simulink model "Assignment2"  (R2021a)
settings: Solver=FixedStepAuto  StartTime=0.0  StopTime=2  FixedStep=1e-3  RelTol=1e-3  EnableMultiTasking=on
undefined symbols (not defined in the file): D0, D1, D10, D11, D12, D13, D2, D3, D4, D5, D6, D7, D8, D9, magnitude, PTA0, PTA1, PTA2, PTB23, PTB9, PTC16, PTC17, PTC2, PTC3, PTC4, PTD0, PTD1, PTD2, PTD3
libraries: frdmk64flib x19, dspstat3 x1
settings Model: EnablePacing=on  PacingRate=0.250000  ExtModeTrigDuration=5  Creator=Arun Mistry  LastModifiedBy=majet
settings OptimizationCC: EnhancedBackFolding=on  PassReuseOutputArgsAs=Individual arguments  ZeroExternalMemoryAtStartup=off  ZeroInternalMemoryAtStartup=off  MaxStackSize=64  OptimizeBlockOrder=speed  DifferentSizesBufferReuse=on  OptimizationCustomize=off  EfficientTunableParamExpr=on
settings DebuggingCC: ParameterTunabilityLossMsg=error
settings HardwareCC: ProdBitPerPointer=32  ProdBitPerSizeT=32  ProdBitPerPtrDiffT=32  ProdLargestAtomicInteger=Long  ProdLargestAtomicFloat=Double  ProdWordSize=32  ProdHWDeviceType=ARM Compatible->ARM Cortex
settings SFSimCC: MATLABDynamicMemAlloc=off
settings RTWCC: SystemTargetFile=ert.tlc  HardwareBoard=NXP FRDM-K64F  TLCOptions="-aInlineSetEventsForThisBaseRateFcn=TLC_FALSE -aSuppressMultiTaskScheduler=TLC_FALSE  -aRateBasedStepFcn=0"  TemplateMakefile=ert_default_tmf  Toolchain=GNU Tools for ARM Embedded Processors
settings CodeAppCC: ForceParamTrailComments=on  IgnoreCustomStorageClasses=off  OperatorAnnotations=on  SimulinkDataObjDesc=on  SFDataObjDesc=on  InsertBlockDesc=on
settings ERTTargetCC: ExtModeTransport=4  ExtModeMexFile=sendToCommService

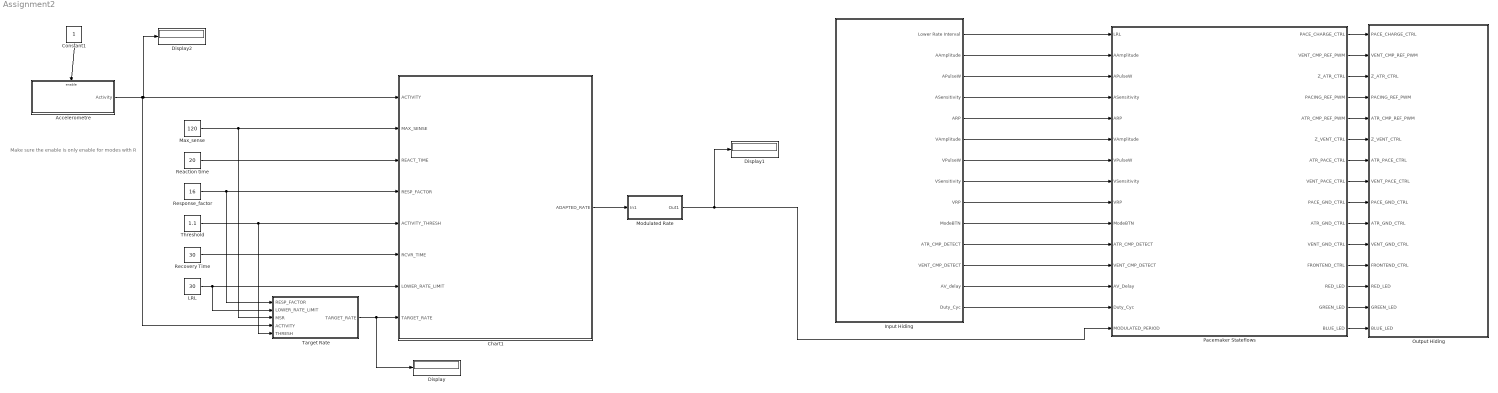
== system Assignment2 ==
  note: Make sure the enable is only enable for modes with R
  Accelerometre : Subsystem
  Chart1 : Stateflow chart  TreatAsAtomicUnit=on
  Constant1 : Constant  OutDataTypeStr=uint16
  Display : Display
  Display1 : Display
  Display2 : Display
  Input Hiding : Subsystem
  LRL : Constant  Value=30  OutDataTypeStr=uint16
  Max_sense : Constant  Value=120  OutDataTypeStr=uint16
  Modulated Rate : Subsystem
  Output Hiding : Subsystem
  Pacemaker Stateflows : Stateflow chart  TreatAsAtomicUnit=on
      settings: PortSchema="{\"entries\":[{\"content\":{\"sides\":[{\"content\":{\"connectorIds\":[\"In1\",\"In2\",\"In3\",\"In4\",\"In5\",\"In6\",\"In7\",\"In8\",\"In9\",\"In10\",\"In11\",\"In12\",\"In13\",\"In15\",\"In14\"]},\"type\":\"ConnectorPlacement.EquallySpacedRectSide\",\"uuid\":\"73ec282f-bdc5-469f-8e6f-a94c3bdc9020\"},{\"content\":{\"connectorIds\":[\"Out1\",\"Out2\",\"Out3\",\"Out4\",\"Out5\",\"Out6\",\"Out7\",\"Out8\",\"Out9\",\"Out10\",\"Out11\",\"Out12\",\"Out13\",\"Out14\",\"Out15\"],\"side\":\"RIGHT\"},\"type\":\"ConnectorPlacement.EquallySpacedRectSide\",\"uuid\":\"8dd20006-a4c5-4baa-83a8-987332cd4bb4\"},{\"content\":{\"connectorIds\":[],\"side\":\"TOP\"},\"type\":\"ConnectorPlacement.EquallySpacedRectSide\",\"uuid\":\"22935e9b-efaa-43e1-8cc8-2e08fa14d9a6\"},{\"content\":{\"connectorIds\":[],\"side\":\"BOTTOM\"},\"type\":\"ConnectorPlacement.EquallySpacedRectSide\",\"uuid\":\"9851d334-d076-4ac0-89c9-77644970121a\"}]},\"type\":\"ConnectorPlacement.EquallySpacedConnector\",\"uuid\":\"2847227f-03fa-454f-95d6-41e472bd469d\"}],\"packageUris\":[\"http://schema.mathworks.com/mf0/Connector/R2020b\"],\"version\":\"1.0\"}"
  Reaction time : Constant  Value=20  OutDataTypeStr=uint16
  Recovery Time : Constant  Value=30  OutDataTypeStr=uint16
  Response_factor : Constant  Value=16  OutDataTypeStr=uint16
  Target Rate : Subsystem
  Threshold : Constant  Value=1.1  OutDataTypeStr=double
  wires:
  Pacemaker Stateflows/1(PACE_CHARGE_CTRL) -> Output Hiding/1(PACE_CHARGE_CTRL)
  Input Hiding/11(ATR_CMP_DETECT) -> Pacemaker Stateflows/11(ATR_CMP_DETECT)
  Input Hiding/7(VPulseW) -> Pacemaker Stateflows/7(VPulseW)
  Input Hiding/12(VENT_CMP_DETECT) -> Pacemaker Stateflows/12(VENT_CMP_DETECT)
  Pacemaker Stateflows/3(Z_ATR_CTRL) -> Output Hiding/3(Z_ATR_CTRL)
  Input Hiding/3(APulseW) -> Pacemaker Stateflows/3(APulseW)
  Pacemaker Stateflows/7(ATR_PACE_CTRL) -> Output Hiding/7(ATR_PACE_CTRL)
  Pacemaker Stateflows/10(ATR_GND_CTRL) -> Output Hiding/10(ATR_GND_CTRL)
  Input Hiding/10(ModeBTN) -> Pacemaker Stateflows/10(ModeBTN)
  Input Hiding/2(AAmplitude) -> Pacemaker Stateflows/2(AAmplitude)
  Input Hiding/6(VAmplitude) -> Pacemaker Stateflows/6(VAmplitude)
  Pacemaker Stateflows/6(Z_VENT_CTRL) -> Output Hiding/6(Z_VENT_CTRL)
  Pacemaker Stateflows/4(PACING_REF_PWM) -> Output Hiding/4(PACING_REF_PWM)
  Pacemaker Stateflows/11(VENT_GND_CTRL) -> Output Hiding/11(VENT_GND_CTRL)
  Pacemaker Stateflows/9(PACE_GND_CTRL) -> Output Hiding/9(PACE_GND_CTRL)
  Pacemaker Stateflows/8(VENT_PACE_CTRL) -> Output Hiding/8(VENT_PACE_CTRL)
  Input Hiding/1(Lower Rate Interval) -> Pacemaker Stateflows/1(LRL)
  Pacemaker Stateflows/15(BLUE_LED) -> Output Hiding/15(BLUE_LED)
  Input Hiding/4(ASensitivity) -> Pacemaker Stateflows/4(ASensitivity)
  Pacemaker Stateflows/12(FRONTEND_CTRL) -> Output Hiding/12(FRONTEND_CTRL)
  Input Hiding/9(VRP) -> Pacemaker Stateflows/9(VRP)
  Input Hiding/8(VSensitivity) -> Pacemaker Stateflows/8(VSensitivity)
  Input Hiding/5(ARP) -> Pacemaker Stateflows/5(ARP)
  Pacemaker Stateflows/14(GREEN_LED) -> Output Hiding/14(GREEN_LED)
  Pacemaker Stateflows/13(RED_LED) -> Output Hiding/13(RED_LED)
  Pacemaker Stateflows/5(ATR_CMP_REF_PWM) -> Output Hiding/5(ATR_CMP_REF_PWM)
  Pacemaker Stateflows/2(VENT_CMP_REF_PWM) -> Output Hiding/2(VENT_CMP_REF_PWM)
  Input Hiding/14(Duty_Cyc) -> Pacemaker Stateflows/15(Duty_Cyc)
  LRL/1 -> Target Rate/2(LOWER_RATE_LIMIT), Chart1/7(LOWER_RATE_LIMIT)
  Chart1/1(ADAPTED_RATE) -> Modulated Rate/1(In1)
  Recovery Time/1 -> Chart1/6(RCVR_TIME)
  Max_sense/1 -> Target Rate/3(MSR), Chart1/2(MAX_SENSE)
  Reaction time/1 -> Chart1/3(REACT_TIME)
  Response_factor/1 -> Target Rate/1(RESP_FACTOR), Chart1/4(RESP_FACTOR)
  Threshold/1 -> Target Rate/5(THRESH), Chart1/5(ACTIVITY_THRESH)
  Modulated Rate/1(Out1) -> Display1/1, Pacemaker Stateflows/14(MODULATED_PERIOD)
  Constant1/1 -> Accelerometre/Enable
  Input Hiding/13(AV_delay) -> Pacemaker Stateflows/13(AV_Delay)
  Target Rate/1(TARGET_RATE) -> Display/1, Chart1/8(TARGET_RATE)
  Accelerometre/1(Activity) -> Target Rate/4(ACTIVITY), Chart1/1(ACTIVITY), Display2/1

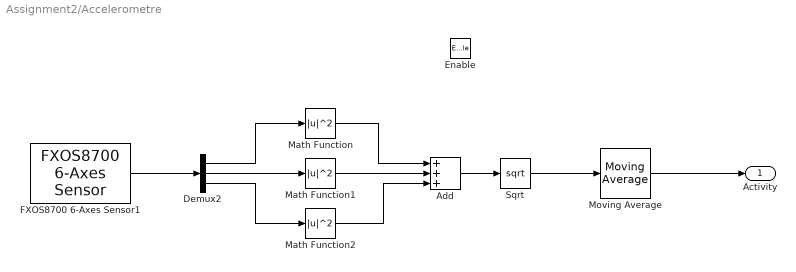
== system Assignment2/Accelerometre ==
  Enable : EnablePort
  Add : Sum  Inputs=+++
  Demux2 : Demux  Outputs=3
  FXOS8700 6-Axes Sensor1 : frdmk64flib/FXOS8700 6-Axes Sensor  Activesensor=Accelerometer only  ODR=100Hz  HybridODR=400Hz  Accelfullrange=-4g to +4g  SampleTime=1/100
  Math Function : Math  Operator=magnitude^2  SignedPower=on  OutDataTypeStr=double  SaturateOnIntegerOverflow=on
  Math Function1 : Math  Operator=magnitude^2  SignedPower=on  OutDataTypeStr=double  SaturateOnIntegerOverflow=on
  Math Function2 : Math  Operator=magnitude^2  SignedPower=on  OutDataTypeStr=double  SaturateOnIntegerOverflow=on
  Moving Average : dspstat3/Moving Average  Method=Sliding window  ForgettingFactorPort=off  SpecifyWindowLength=on  WindowLength=4  ForgettingFactor=0.9  SimulateUsing=Code generation
  Sqrt : Sqrt  SaturateOnIntegerOverflow=on
  Activity : Outport  OutDataTypeStr=double  SourceOfInitialOutputValue=Input signal
  wires:
  Sqrt/1 -> Moving Average/1
  FXOS8700 6-Axes Sensor1/1 -> Demux2/1
  Math Function/1 -> Add/1
  Add/1 -> Sqrt/1
  Math Function2/1 -> Add/3
  Demux2/2 -> Math Function1/1
  Math Function1/1 -> Add/2
  Demux2/1 -> Math Function/1
  Demux2/3 -> Math Function2/1
  Moving Average/1 -> Activity/1

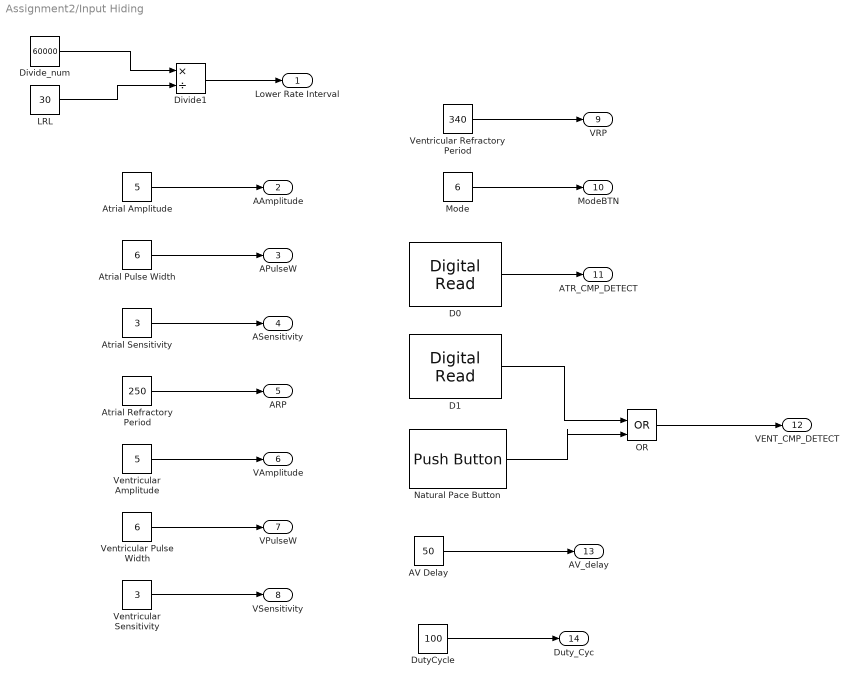
== system Assignment2/Input Hiding ==
  AV Delay : Constant  Value=50  OutDataTypeStr=uint16
  Atrial Amplitude : Constant  Value=5  OutDataTypeStr=uint16
  Atrial Pulse Width : Constant  Value=6  OutDataTypeStr=uint16
  Atrial Refractory Period : Constant  Value=250  OutDataTypeStr=uint16
  Atrial Sensitivity : Constant  Value=3  OutDataTypeStr=uint16
  D0 : frdmk64flib/Digital Read  Whichpin=PTC16 (D0)  SampleTime=-1
  D1 : frdmk64flib/Digital Read  Whichpin=PTC17 (D1)  SampleTime=-1
  Divide1 : Product  Inputs=*/  OutDataTypeStr=uint16  RndMeth=Round
  Divide_num : Constant  Value=60000  OutDataTypeStr=uint16
  DutyCycle : Constant  Value=100  OutDataTypeStr=uint16
  LRL : Constant  Value=30  OutDataTypeStr=uint16
  Mode : Constant  Value=6  OutDataTypeStr=uint16
  Natural Pace Button : frdmk64flib/Push Button  Whichswitch=SW3  SampleTime1=-1
  OR : Logic  Operator=OR  IconShape=distinctive  AllPortsSameDT=off  OutDataTypeStr=boolean
  Ventricular Amplitude : Constant  Value=5  OutDataTypeStr=uint16
  Ventricular Pulse Width : Constant  Value=6  OutDataTypeStr=uint16
  Ventricular Refractory Period : Constant  Value=340  OutDataTypeStr=uint16
  Ventricular Sensitivity : Constant  Value=3  OutDataTypeStr=uint16
  Lower Rate Interval : Outport  OutDataTypeStr=uint16
  AAmplitude : Outport  Port=2  OutDataTypeStr=uint16
  APulseW : Outport  Port=3  OutDataTypeStr=uint16
  ASensitivity : Outport  Port=4  OutDataTypeStr=uint16
  ARP : Outport  Port=5  OutDataTypeStr=uint16
  VAmplitude : Outport  Port=6  OutDataTypeStr=uint16
  VPulseW : Outport  Port=7  OutDataTypeStr=uint16
  VSensitivity : Outport  Port=8  OutDataTypeStr=uint16
  VRP : Outport  Port=9  OutDataTypeStr=uint16
  ModeBTN : Outport  Port=10  OutDataTypeStr=uint16
  ATR_CMP_DETECT : Outport  Port=11  OutDataTypeStr=boolean
  VENT_CMP_DETECT : Outport  Port=12  OutDataTypeStr=boolean
  AV_delay : Outport  Port=13  OutDataTypeStr=uint16
  Duty_Cyc : Outport  Port=14  OutDataTypeStr=uint16
  wires:
  Atrial Amplitude/1 -> AAmplitude/1
  Ventricular Amplitude/1 -> VAmplitude/1
  Atrial Pulse Width/1 -> APulseW/1
  Ventricular Pulse Width/1 -> VPulseW/1
  Atrial Sensitivity/1 -> ASensitivity/1
  Ventricular Sensitivity/1 -> VSensitivity/1
  Ventricular Refractory Period/1 -> VRP/1
  Atrial Refractory Period/1 -> ARP/1
  D0/1 -> ATR_CMP_DETECT/1
  Natural Pace Button/1 -> OR/2
  Mode/1 -> ModeBTN/1
  DutyCycle/1 -> Duty_Cyc/1
  Divide_num/1 -> Divide1/1
  Divide1/1 -> Lower Rate Interval/1
  D1/1 -> OR/1
  OR/1 -> VENT_CMP_DETECT/1
  AV Delay/1 -> AV_delay/1
  LRL/1 -> Divide1/2

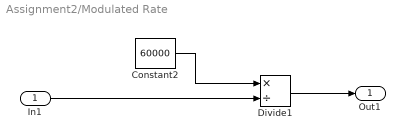
== system Assignment2/Modulated Rate ==
  In1 : Inport  OutDataTypeStr=uint16
  Constant2 : Constant  Value=60000  OutDataTypeStr=uint16
  Divide1 : Product  Inputs=*/  OutDataTypeStr=uint16
  Out1 : Outport  OutDataTypeStr=uint16
  wires:
  In1/1 -> Divide1/2
  Constant2/1 -> Divide1/1
  Divide1/1 -> Out1/1

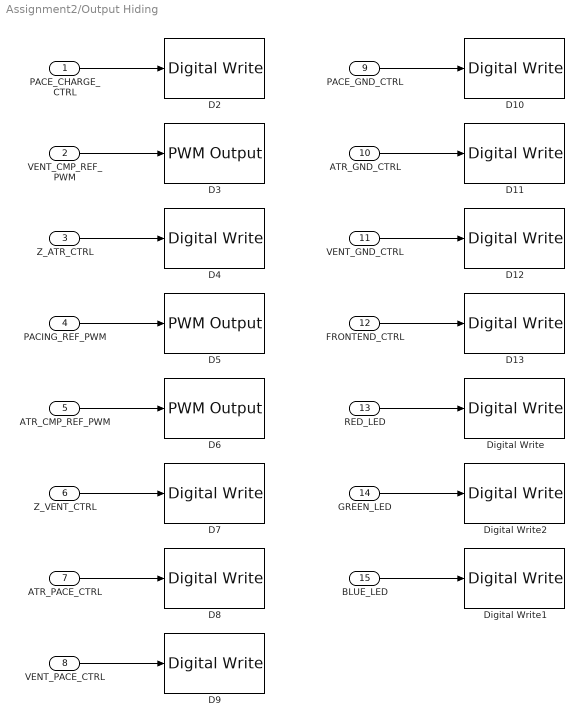
== system Assignment2/Output Hiding ==
  PACE_CHARGE_CTRL : Inport  OutDataTypeStr=uint16
  VENT_CMP_REF_PWM : Inport  Port=2  OutDataTypeStr=uint16
  Z_ATR_CTRL : Inport  Port=3  OutDataTypeStr=uint16
  PACING_REF_PWM : Inport  Port=4  OutDataTypeStr=uint16
  ATR_CMP_REF_PWM : Inport  Port=5  OutDataTypeStr=uint16
  Z_VENT_CTRL : Inport  Port=6  OutDataTypeStr=uint16
  ATR_PACE_CTRL : Inport  Port=7  OutDataTypeStr=uint16
  VENT_PACE_CTRL : Inport  Port=8  OutDataTypeStr=uint16
  PACE_GND_CTRL : Inport  Port=9  OutDataTypeStr=uint16
  ATR_GND_CTRL : Inport  Port=10  OutDataTypeStr=uint16
  VENT_GND_CTRL : Inport  Port=11  OutDataTypeStr=uint16
  FRONTEND_CTRL : Inport  Port=12  OutDataTypeStr=uint16
  RED_LED : Inport  Port=13  OutDataTypeStr=uint16
  GREEN_LED : Inport  Port=14  OutDataTypeStr=uint16
  BLUE_LED : Inport  Port=15  OutDataTypeStr=uint16
  D10 : frdmk64flib/Digital Write  Whichpin=PTD0 (D10)
  D11 : frdmk64flib/Digital Write  Whichpin=PTD2 (D11)
  D12 : frdmk64flib/Digital Write  Whichpin=PTD3 (D12)
  D13 : frdmk64flib/Digital Write  Whichpin=PTD1 (D13)
  D2 : frdmk64flib/Digital Write  Whichpin=PTB9 (D2)
  D3 : frdmk64flib/PWM Output  Whichpin=PTA1 (D3)  InitialFrequency=2000  InitialDutyCycle=100
  D4 : frdmk64flib/Digital Write  Whichpin=PTB23 (D4)
  D5 : frdmk64flib/PWM Output  Whichpin=PTA2 (D5)  InitialFrequency=2000  InitialDutyCycle=100
  D6 : frdmk64flib/PWM Output  Whichpin=PTC2 (D6)  InitialFrequency=2000  InitialDutyCycle=100
  D7 : frdmk64flib/Digital Write  Whichpin=PTC3 (D7)
  "D8 " : frdmk64flib/Digital Write  Whichpin=PTA0 (D8)
  D9 : frdmk64flib/Digital Write  Whichpin=PTC4 (D9)
  Digital Write : frdmk64flib/Digital Write  Whichpin=RED_LED
  Digital Write1 : frdmk64flib/Digital Write  Whichpin=BLUE_LED
  Digital Write2 : frdmk64flib/Digital Write  Whichpin=GREEN_LED
  wires:
  VENT_PACE_CTRL/1 -> D9/1
  ATR_CMP_REF_PWM/1 -> D6/1
  PACE_GND_CTRL/1 -> D10/1
  VENT_CMP_REF_PWM/1 -> D3/1
  PACING_REF_PWM/1 -> D5/1
  ATR_GND_CTRL/1 -> D11/1
  ATR_PACE_CTRL/1 -> "D8 "/1
  PACE_CHARGE_CTRL/1 -> D2/1
  FRONTEND_CTRL/1 -> D13/1
  VENT_GND_CTRL/1 -> D12/1
  Z_ATR_CTRL/1 -> D4/1
  Z_VENT_CTRL/1 -> D7/1
  RED_LED/1 -> Digital Write/1
  BLUE_LED/1 -> Digital Write1/1
  GREEN_LED/1 -> Digital Write2/1

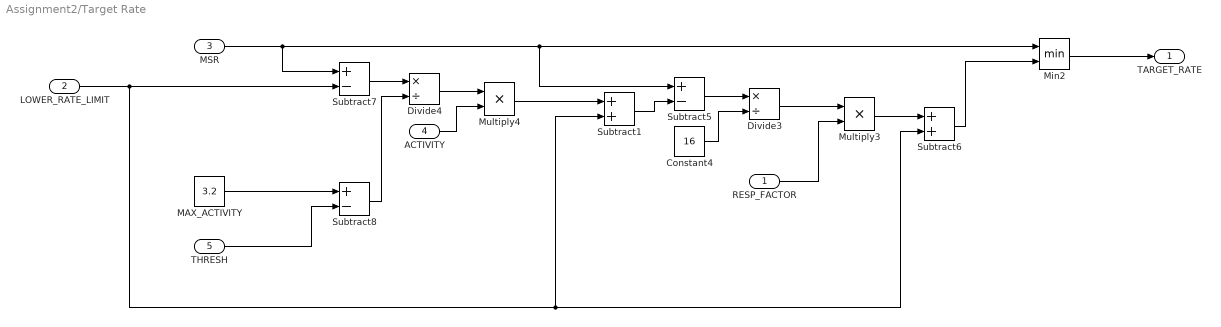
== system Assignment2/Target Rate ==
  RESP_FACTOR : Inport  OutDataTypeStr=uint16
  LOWER_RATE_LIMIT : Inport  Port=2  OutDataTypeStr=uint16
  MSR : Inport  Port=3  OutDataTypeStr=uint16
  ACTIVITY : Inport  Port=4  OutDataTypeStr=double
  THRESH : Inport  Port=5  OutDataTypeStr=double
  Constant4 : Constant  Value=16  OutDataTypeStr=double
  Divide3 : Product  Inputs=*/  OutDataTypeStr=uint16
  Divide4 : Product  Inputs=*/  OutDataTypeStr=uint16
  MAX_ACTIVITY : Constant  Value=3.2  OutDataTypeStr=double
  Min2 : MinMax  Inputs=2
  Multiply3 : Product  Inputs=**  OutDataTypeStr=uint16  RndMeth=Ceiling
  Multiply4 : Product  Inputs=**  OutDataTypeStr=uint16  RndMeth=Ceiling
  Subtract1 : Sum  AccumDataTypeStr=uint16
  Subtract5 : Sum  Inputs=+-  AccumDataTypeStr=uint16
  Subtract6 : Sum  AccumDataTypeStr=uint16
  Subtract7 : Sum  Inputs=+-  AccumDataTypeStr=uint16
  Subtract8 : Sum  Inputs=+-  AccumDataTypeStr=double
  TARGET_RATE : Outport  OutDataTypeStr=uint16  SourceOfInitialOutputValue=Input signal
  wires:
  MSR/1 -> Subtract5/1, Min2/1, Subtract7/1
  ACTIVITY/1 -> Multiply4/2
  Constant4/1 -> Divide3/2
  Divide4/1 -> Multiply4/1
  Divide3/1 -> Multiply3/1
  Subtract5/1 -> Divide3/1
  MAX_ACTIVITY/1 -> Subtract8/1
  Subtract6/1 -> Min2/2
  Subtract8/1 -> Divide4/2
  LOWER_RATE_LIMIT/1 -> Subtract7/2, Subtract1/2, Subtract6/2
  THRESH/1 -> Subtract8/2
  Multiply3/1 -> Subtract6/1
  RESP_FACTOR/1 -> Multiply3/2
  Min2/1 -> TARGET_RATE/1
  Subtract7/1 -> Divide4/1
  Subtract1/1 -> Subtract5/2
  Multiply4/1 -> Subtract1/1

== stateflow chart Assignment2/Pacemaker Stateflows ==
  state MODE_CHOOSE
  state AOO
    entry:
    VENT_PACE_CTRL = 0; VENT_GND_CTRL = 0; PACE_GND_CTRL = 1; Z_VENT_CTRL = 0;
    Z_ATR_CTRL = 0;ATR_PACE_CTRL = 0; PACING_REF_PWM = Duty_Cyc;
    state PACE_ATR
      entry:
      PACE_CHARGE_CTRL = 0;
      ATR_GND_CTRL = 0;
      ATR_PACE_CTRL = 1;
      RED_LED = 1;
    state C22_CHARGE
      entry:
      PACE_CHARGE_CTRL = 1;
      ATR_PACE_CTRL = 0;
      ATR_GND_CTRL = 1;
      RED_LED = 0;
    (default) -> AOO.C22_CHARGE
    AOO.PACE_ATR -> AOO.C22_CHARGE : after(APulseW,msec)
    AOO.C22_CHARGE -> AOO.PACE_ATR : after(LRL-APulseW,msec)
  state AOOR
    entry:
    VENT_PACE_CTRL = 0; VENT_GND_CTRL = 0; PACE_GND_CTRL = 1; Z_VENT_CTRL = 0;
    Z_ATR_CTRL = 0;ATR_PACE_CTRL = 0; PACING_REF_PWM = Duty_Cyc;
    state C22_CHARGE
      entry:
      PACE_CHARGE_CTRL = 1;
      ATR_PACE_CTRL = 0;
      ATR_GND_CTRL = 1;
      RED_LED = 0;
    state PACE_ATR
      entry:
      PACE_CHARGE_CTRL = 0;
      ATR_GND_CTRL = 0;
      ATR_PACE_CTRL = 1;
      RED_LED = 1;
    (default) -> AOOR.PACE_ATR
    AOOR.PACE_ATR -> AOOR.C22_CHARGE : after(APulseW,msec)
    AOOR.C22_CHARGE -> AOOR.PACE_ATR : after(MODULATED_PERIOD-APulseW,msec)
  state AAI
    entry:
    VENT_PACE_CTRL = 0; VENT_GND_CTRL = 0; ATR_CMP_REF_PWM = 70;
    Z_VENT_CTRL = 0; Z_ATR_CTRL = 0;PACING_REF_PWM = Duty_Cyc;PACE_GND_CTRL = 1;FRONTEND_CTRL = 1; sense = 0;
    state C22_CHARGE
      entry:
      RED_LED = 0;
      PACE_CHARGE_CTRL = 1;
      ATR_GND_CTRL = 1;
      ATR_PACE_CTRL = 0;
      sense = 0;
    state PACE_ATR
      entry:
      RED_LED = 1;
      PACE_CHARGE_CTRL = 0;
      ATR_GND_CTRL = 0;
      ATR_PACE_CTRL = 1;
      sense = 1;
    state REFRACTORY
      entry:
      GREEN_LED = 1;
      PACE_CHARGE_CTRL = 1;
      ATR_GND_CTRL = 1;
      ATR_PACE_CTRL = 0;
    (default) -> AAI.C22_CHARGE
    AAI.REFRACTORY -> AAI.C22_CHARGE : after(ARP-(APulseW * sense),msec)
    AAI.C22_CHARGE -> AAI.PACE_ATR [order 2] : after(LRL-ARP,msec)
    AAI.PACE_ATR -> AAI.REFRACTORY : after(APulseW,msec)
    AAI.C22_CHARGE -> AAI.REFRACTORY [order 1] : [ATR_CMP_DETECT == true]
  state AAIR
    entry:
    VENT_PACE_CTRL = 0; VENT_GND_CTRL = 0; ATR_CMP_REF_PWM = 70;
    Z_VENT_CTRL = 0; Z_ATR_CTRL = 0;PACING_REF_PWM = Duty_Cyc;PACE_GND_CTRL = 1;FRONTEND_CTRL = 1; sense = 0;
    state C22_CHARGE
      entry:
      RED_LED = 0;
      PACE_CHARGE_CTRL = 1;
      ATR_GND_CTRL = 1;
      ATR_PACE_CTRL = 0;
      sense = 0;
    state PACE_ATR
      entry:
      RED_LED = 1;
      PACE_CHARGE_CTRL = 0;
      ATR_GND_CTRL = 0;
      ATR_PACE_CTRL = 1;
      sense = 1;
    state REFRACTORY
      entry:
      GREEN_LED = 1;
      PACE_CHARGE_CTRL = 1;
      ATR_GND_CTRL = 1;
      ATR_PACE_CTRL = 0;
    (default) -> AAIR.C22_CHARGE
    AAIR.REFRACTORY -> AAIR.C22_CHARGE : after(ARP-(APulseW * sense),msec)
    AAIR.C22_CHARGE -> AAIR.PACE_ATR [order 2] : after(MODULATED_PERIOD-ARP,msec)
    AAIR.PACE_ATR -> AAIR.REFRACTORY : after(APulseW,msec)
    AAIR.C22_CHARGE -> AAIR.REFRACTORY [order 1] : [ATR_CMP_DETECT == true]
  state VOO
    entry:
    ATR_PACE_CTRL = 0; ATR_GND_CTRL = 0; PACE_GND_CTRL = 1;
    Z_ATR_CTRL = 0; Z_VENT_CTRL = 0; PACING_REF_PWM = Duty_Cyc;
    state PACE_VENT
      entry:
      PACE_CHARGE_CTRL = 0;
      VENT_GND_CTRL = 0;
      VENT_PACE_CTRL = 1;
      BLUE_LED = 1;
    state C22_CHARGE
      entry:
      VENT_PACE_CTRL = 0;
      VENT_GND_CTRL = 1;
      PACE_CHARGE_CTRL = 1;
      BLUE_LED = 0;
    (default) -> VOO.C22_CHARGE
    VOO.PACE_VENT -> VOO.C22_CHARGE : after(VPulseW,msec)
    VOO.C22_CHARGE -> VOO.PACE_VENT : after(LRL-VPulseW,msec)
  state VOOR
    entry:
    ATR_PACE_CTRL = 0; ATR_GND_CTRL = 0; PACE_GND_CTRL = 1;
    Z_ATR_CTRL = 0; Z_VENT_CTRL = 0; PACING_REF_PWM = Duty_Cyc;
    state PACE_VENT
      entry:
      PACE_CHARGE_CTRL = 0;
      VENT_GND_CTRL = 0;
      VENT_PACE_CTRL = 1;
      BLUE_LED = 1;
    state C22_CHARGE
      entry:
      VENT_PACE_CTRL = 0;
      VENT_GND_CTRL = 1;
      PACE_CHARGE_CTRL = 1;
      BLUE_LED = 0;
    (default) -> VOOR.C22_CHARGE
    VOOR.PACE_VENT -> VOOR.C22_CHARGE : after(VPulseW,msec)
    VOOR.C22_CHARGE -> VOOR.PACE_VENT : after(MODULATED_PERIOD-VPulseW,msec)
  state VVI
    entry:
    ATR_PACE_CTRL = 0; ATR_GND_CTRL = 0; PACE_GND_CTRL = 1; VENT_CMP_REF_PWM = 70;
    Z_VENT_CTRL = 0; Z_ATR_CTRL = 0;FRONTEND_CTRL = 1; PACING_REF_PWM = Duty_Cyc; sense = 0;
    state PACE_VENT
      entry:
      BLUE_LED = 1;
      PACE_CHARGE_CTRL = 0;
      VENT_GND_CTRL = 0;
      VENT_PACE_CTRL = 1;
      sense = 1;
    state C22_CHARGE
      entry:
      BLUE_LED = 0;
      PACE_CHARGE_CTRL = 1;
      VENT_GND_CTRL = 1;
      VENT_PACE_CTRL = 0;
      sense = 0;
    state REFRACTORY
      entry:
      GREEN_LED = 1;
      PACE_CHARGE_CTRL = 1;
      VENT_GND_CTRL = 1;
      VENT_PACE_CTRL = 0;
    (default) -> VVI.C22_CHARGE
    VVI.C22_CHARGE -> VVI.PACE_VENT [order 2] : after(LRL-VRP,msec)
    VVI.REFRACTORY -> VVI.C22_CHARGE : after(VRP-(VPulseW *sense),msec)
    VVI.PACE_VENT -> VVI.REFRACTORY : after(VPulseW,msec)
    VVI.C22_CHARGE -> VVI.REFRACTORY [order 1] : [VENT_CMP_DETECT == true]
  state VVIR
    entry:
    ATR_PACE_CTRL = 0; ATR_GND_CTRL = 0; PACE_GND_CTRL = 1; VENT_CMP_REF_PWM = 70;
    Z_VENT_CTRL = 0; Z_ATR_CTRL = 0;FRONTEND_CTRL = 1; PACING_REF_PWM = Duty_Cyc; sense = 0;
    state PACE_VENT
      entry:
      BLUE_LED = 1;
      PACE_CHARGE_CTRL = 0;
      VENT_GND_CTRL = 0;
      VENT_PACE_CTRL = 1;
      sense = 1;
    state C22_CHARGE
      entry:
      BLUE_LED = 0;
      PACE_CHARGE_CTRL = 1;
      VENT_GND_CTRL = 1;
      VENT_PACE_CTRL = 0;
      sense = 0;
    state REFRACTORY
      entry:
      GREEN_LED = 1;
      PACE_CHARGE_CTRL = 1;
      VENT_GND_CTRL = 1;
      VENT_PACE_CTRL = 0;
    (default) -> VVIR.C22_CHARGE
    VVIR.C22_CHARGE -> VVIR.PACE_VENT [order 2] : after(MODULATED_PERIOD-VRP,msec)
    VVIR.REFRACTORY -> VVIR.C22_CHARGE : after(VRP-(VPulseW *sense),msec)
    VVIR.PACE_VENT -> VVIR.REFRACTORY : after(VPulseW,msec)
    VVIR.C22_CHARGE -> VVIR.REFRACTORY [order 1] : [VENT_CMP_DETECT == true]
  state DOO
    entry:
    Z_VENT_CTRL = 0; Z_ATR_CTRL = 0; PACE_GND_CTRL = 1;
    state C22_CHARGE
      entry:
      ATR_PACE_CTRL = 0;
      VENT_PACE_CTRL = 0;
      PACING_REF_PWM = AAmplitude*20;
      PACE_CHARGE_CTRL = 1;
      ATR_GND_CTRL = 0;
      VENT_GND_CTRL = 1;
      BLUE_LED = 0;
    state PACE_ATR
      entry:
      PACE_CHARGE_CTRL = 0;
      ATR_GND_CTRL = 0;
      VENT_GND_CTRL = 0;
      ATR_PACE_CTRL = 1;
      RED_LED = 1;
    state AV_DELAY_PERIOD
      entry:
      ATR_PACE_CTRL = 0;
      VENT_PACE_CTRL = 0;
      PACING_REF_PWM = VAmplitude*20;
      PACE_CHARGE_CTRL = 1;
      ATR_GND_CTRL = 1;
      VENT_GND_CTRL = 0;
      RED_LED = 0;
      BLUE_LED = 0;
    state PACE_VENT
      entry:
      PACE_CHARGE_CTRL = 0;
      ATR_GND_CTRL = 0;
      VENT_GND_CTRL = 0;
      VENT_PACE_CTRL = 1;
      BLUE_LED = 1;
    (default) -> DOO.C22_CHARGE
    DOO.C22_CHARGE -> DOO.PACE_ATR : after(LRL-AV_Delay-VPulseW,msec)
    DOO.PACE_ATR -> DOO.AV_DELAY_PERIOD : after(APulseW,msec)
    DOO.PACE_VENT -> DOO.C22_CHARGE : after(VPulseW, msec)
    DOO.AV_DELAY_PERIOD -> DOO.PACE_VENT : after(AV_Delay-APulseW,msec)
  state DOOR
    entry:
    Z_VENT_CTRL = 0; Z_ATR_CTRL = 0; PACE_GND_CTRL = 1;
    state C22_CHARGE
      entry:
      ATR_PACE_CTRL = 0;
      VENT_PACE_CTRL = 0;
      PACING_REF_PWM = AAmplitude*20;
      PACE_CHARGE_CTRL = 1;
      ATR_GND_CTRL = 0;
      VENT_GND_CTRL = 1;
      BLUE_LED = 0;
    state PACE_ATR
      entry:
      PACE_CHARGE_CTRL = 0;
      ATR_GND_CTRL = 0;
      VENT_GND_CTRL = 0;
      ATR_PACE_CTRL = 1;
      RED_LED = 1;
    state AV_DELAY_PERIOD
      entry:
      ATR_PACE_CTRL = 0;
      VENT_PACE_CTRL = 0;
      PACING_REF_PWM = VAmplitude*20;
      PACE_CHARGE_CTRL = 1;
      ATR_GND_CTRL = 1;
      VENT_GND_CTRL = 0;
      RED_LED = 0;
      BLUE_LED = 0;
    state PACE_VENT
      entry:
      PACE_CHARGE_CTRL = 0;
      ATR_GND_CTRL = 0;
      VENT_GND_CTRL = 0;
      VENT_PACE_CTRL = 1;
      BLUE_LED = 1;
    (default) -> DOOR.C22_CHARGE
    DOOR.C22_CHARGE -> DOOR.PACE_ATR : after(MODULATED_PERIOD-AV_Delay-VPulseW,msec)
    DOOR.PACE_ATR -> DOOR.AV_DELAY_PERIOD : after(APulseW,msec)
    DOOR.PACE_VENT -> DOOR.C22_CHARGE : after(VPulseW, msec)
    DOOR.AV_DELAY_PERIOD -> DOOR.PACE_VENT : after(AV_Delay-APulseW,msec)
  MODE_CHOOSE -> AOO [order 5] : [ModeBTN==1]
  (default) -> MODE_CHOOSE
  AOO -> MODE_CHOOSE : [ModeBTN~=1]
  MODE_CHOOSE -> AOOR [order 4] : [ModeBTN==6]
  AOOR -> MODE_CHOOSE : [ModeBTN~=6]
  MODE_CHOOSE -> AAI [order 10] : [ModeBTN==2]
  AAI -> MODE_CHOOSE : [ModeBTN~=2]
  MODE_CHOOSE -> AAIR [order 3] : [ModeBTN==7]
  AAIR -> MODE_CHOOSE : [ModeBTN~=7]
  MODE_CHOOSE -> VOO [order 2] : [ModeBTN==3]
  VOO -> MODE_CHOOSE : [ModeBTN~=3]
  MODE_CHOOSE -> VOOR [order 9] : [ModeBTN==8]
  VOOR -> MODE_CHOOSE : [ModeBTN~=8]
  MODE_CHOOSE -> VVI [order 1] : [ModeBTN==4]
  VVI -> MODE_CHOOSE : [ModeBTN~=4]
  MODE_CHOOSE -> VVIR [order 8] : [ModeBTN==9]
  VVIR -> MODE_CHOOSE : [ModeBTN~=9]
  MODE_CHOOSE -> DOO [order 7] : [ModeBTN==5]
  DOO -> MODE_CHOOSE : [ModeBTN~=5]
  MODE_CHOOSE -> DOOR [order 6] : [ModeBTN==10]
  DOOR -> MODE_CHOOSE : [ModeBTN~=10]
  data: LRL input uint16; AAmplitude input uint16; APulseW input uint16; ASensitivity input uint16; ARP input uint16; VAmplitude input uint16; VPulseW input uint16; VSensitivity input uint16; VRP input uint16; PACE_CHARGE_CTRL output uint16; VENT_CMP_REF_PWM output uint16; Z_ATR_CTRL output uint16; PACING_REF_PWM output uint16; ATR_CMP_REF_PWM output uint16; Z_VENT_CTRL output uint16; ATR_PACE_CTRL output uint16; VENT_PACE_CTRL output uint16; PACE_GND_CTRL output uint16; ATR_GND_CTRL output uint16; VENT_GND_CTRL output uint16; ModeBTN input uint16; FRONTEND_CTRL output uint16; RED_LED output uint16; GREEN_LED output uint16; BLUE_LED output uint16; ATR_CMP_DETECT input boolean; VENT_CMP_DETECT input boolean; AV_Delay input uint16; MODULATED_PERIOD input uint16; Duty_Cyc input uint16; sense local uint16; pace local uint16

== stateflow chart Assignment2/Chart1 ==
  state STEP_UP
    ADAPTED_RATE = ADAPTED_RATE + ((TARGET_RATE - LOWER_RATE_LIMIT) / (REACT_TIME));
  state MAX
    ADAPTED_RATE = MAX_SENSE
  state STEP_DOWN
    ADAPTED_RATE = ADAPTED_RATE - ((TARGET_RATE - LOWER_RATE_LIMIT) / (RCVR_TIME ));
  state INIT
    entry:
    ADAPTED_RATE = LOWER_RATE_LIMIT
  state MIN
    ADAPTED_RATE = LOWER_RATE_LIMIT
  STEP_UP -> STEP_UP [order 3] : [ACTIVITY > ACTIVITY_THRESH]
  STEP_UP -> MAX [order 1] : [ADAPTED_RATE >= MAX_SENSE]
  INIT -> STEP_UP [order 2] : [ACTIVITY > ACTIVITY_THRESH]
  MIN -> STEP_UP : [ACTIVITY > ACTIVITY_THRESH]
  MAX -> STEP_DOWN : [ACTIVITY <= ACTIVITY_THRESH]
  STEP_UP -> STEP_DOWN [order 2] : [ACTIVITY <= ACTIVITY_THRESH]
  STEP_DOWN -> STEP_UP [order 3] : [ACTIVITY > ACTIVITY_THRESH]
  (default) -> INIT
  STEP_DOWN -> MIN [order 1] : [ADAPTED_RATE <= LOWER_RATE_LIMIT]
  STEP_DOWN -> STEP_DOWN [order 2] : [ACTIVITY <= ACTIVITY_THRESH]
  INIT -> INIT [order 1] : [ACTIVITY <= ACTIVITY_THRESH]
  data: ACTIVITY input double; ADAPTED_RATE output uint16; MAX_SENSE input uint16; REACT_TIME input uint16; RESP_FACTOR input uint16; ACTIVITY_THRESH input double; RCVR_TIME input uint16; LOWER_RATE_LIMIT input uint16; step_up local uint16; step_down local uint16; TARGET_RATE input uint16; TIME local uint16
